simulink model "AnACC_System__impl"  (R2017b)
settings: Solver=FixedStepDiscrete  StartTime=0.0  StopTime=10.0  FixedStep=1  RelTol=1e-3
PreLoadFcn:
  | sl_refresh_customizations
  | enum_Simulink
  | simulinkExportUnitCs
  | ACC_Parameters
  | ACCData
InitFcn:
  | checkUnitMismatch
undefined symbols (not defined in the file): kd, ki, kp, LongRangeRadarUpperLimit, ShortRangeRadarUpperLimit
settings Model: Creator=eh6qym  LastModifiedBy=eh6qym
settings OptimizationCC: DefaultParameterBehavior=Inlined  PassReuseOutputArgsAs=Individual arguments  ZeroExternalMemoryAtStartup=off
settings DebuggingCC: SignalRangeChecking=error  InheritedTsInSrcMsg=none  ParameterTunabilityLossMsg=error
settings SFSimCC: MATLABDynamicMemAlloc=off
settings RTWCC: SystemTargetFile=esd_ert.tlc  GenCodeOnly=on  TemplateMakefile=ert_default_tmf  Description=CSD  GenerateReport=on  IncludeHyperlinkInReport=on  LaunchReport=on  GenerateTraceInfo=on  GenerateTraceReport=on  GenerateTraceReportSl=on  GenerateTraceReportSf=on  GenerateTraceReportEml=on
settings CodeAppCC: ForceParamTrailComments=on  IgnoreCustomStorageClasses=off  OperatorAnnotations=on  SimulinkDataObjDesc=on  SFDataObjDesc=on  InsertBlockDesc=on
settings STFCustomTargetCC: TargetLangStandard=C99 (ISO)  MultiwordLength=256  GenerateSampleERTMain=on  IncludeMdlTerminateFcn=off  CombineOutputUpdateFcns=on  CombineSignalStateStructs=on  SuppressErrorStatus=on  ERTCustomFileBanners=on  MultiInstanceERTCode=on  CodeInterfacePackaging=Reusable function  SupportContinuousTime=off  SupportNonInlinedSFcns=off  RemoveDisableFunc=on  RemoveResetFunc=on  MATLABClassNameForMDSCustomization=Simulink.SoftwareTarget.ERTCustomization  GRTInterface=off  SystemTargetFile=esd_ert.tlc
settings ERTTargetCC: TargetLangStandard=C99 (ISO)  GenerateSampleERTMain=on  ParMdlRefBuildCompliant=off  CompOptLevelCompliant=off  ConcurrentExecutionCompliant=off  IncludeMdlTerminateFcn=off  CombineSignalStateStructs=on  SuppressErrorStatus=on  MultiInstanceERTCode=on  CodeInterfacePackaging=Reusable function  RemoveDisableFunc=on  ModelStepFunctionPrototypeControlCompliant=off  CPPClassGenCompliant=off  UseToolchainInfoCompliant=off  InlinedParameterPlacement=NonHierarchical  ERTCustomFileTemplate=example_file_process.tlc

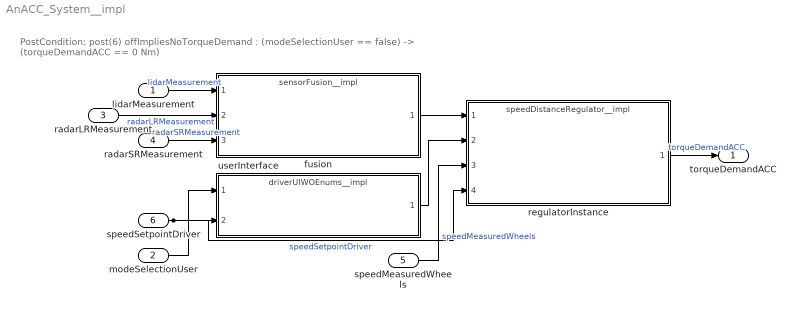
== system AnACC_System__impl ==
  note: PostCondition:
      | post(6) offImpliesNoTorqueDemand :   (modeSelectionUser == false) -> (torqueDemandACC == 0 Nm)
  lidarMeasurement : Inport  OutDataTypeStr=double  Unit=m
      settings: AttributesFormatString=(m)
  modeSelectionUser : Inport  Port=2  OutDataTypeStr=boolean
  radarLRMeasurement : Inport  Port=3  OutDataTypeStr=double  Unit=m
      settings: AttributesFormatString=(m)
  radarSRMeasurement : Inport  Port=4  OutDataTypeStr=double  Unit=cm
      settings: AttributesFormatString=(cm)
  speedMeasuredWheels : Inport  Port=5  OutDataTypeStr=double  Unit=kmh
      settings: AttributesFormatString=(kmh)
  speedSetpointDriver : Inport  Port=6  OutDataTypeStr=double  Unit=kmh
      settings: AttributesFormatString=(kmh)
  fusion : ModelReference  Tag=sensorFusion__impl  ModelNameDialog=sensorFusion__impl  ParameterArgumentNames=LongRangeRadarUpperLimit,ShortRangeRadarUpperLimit  ParameterArgumentValues=LongRangeRadarUpperLimit,ShortRangeRadarUpperLimit  UsingDefaultArgumentValue=0,0  SimulationMode=Normal  ModelReferenceVersion=1.19  LongRangeRadarUpperLimit=RadarRanges.LongRangeRadarUpperLimit  ShortRangeRadarUpperLimit=RadarRanges.ShortRangeRadarUpperLimit  SimulationMode=Normal
  regulatorInstance : ModelReference  Tag=speedDistanceRegulator__impl  ModelNameDialog=speedDistanceRegulator__impl  ParameterArgumentNames=kd,ki,kp  ParameterArgumentValues=kd,ki,kp  UsingDefaultArgumentValue=0,0,0  SimulationMode=Normal  ModelReferenceVersion=1.23  kp=1.0  kd=0.5  ki=0.1  SimulationMode=Normal
  userInterface : ModelReference  ModelNameDialog=driverUIWOEnums__impl  SimulationMode=Normal  ModelReferenceVersion=1.19
  torqueDemandACC : Outport  OutDataTypeStr=double  Unit=Nm
      settings: AttributesFormatString=(Nm)
  wires:
  lidarMeasurement/1 -> fusion/1  "lidarMeasurement"
  modeSelectionUser/1 -> userInterface/1
  radarLRMeasurement/1 -> fusion/2  "radarLRMeasurement"
  radarSRMeasurement/1 -> fusion/3  "radarSRMeasurement"
  speedMeasuredWheels/1 -> regulatorInstance/3  "speedMeasuredWheels"
  speedSetpointDriver/1 -> regulatorInstance/4, userInterface/2  "speedSetpointDriver"
  fusion/1 -> regulatorInstance/1
  regulatorInstance/1 -> torqueDemandACC/1  "torqueDemandACC"
  userInterface/1 -> regulatorInstance/2
